simulink library "EOM"  (R2016b)
settings: Solver=VariableStepAuto  StartTime=0.0  StopTime=10.0  RelTol=1e-3
libraries: aerolib6dof2 x1
settings Model: Creator=Andrew  LastModifiedBy=Andrew

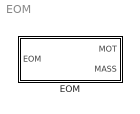
== system EOM ==
  EOM : Subsystem

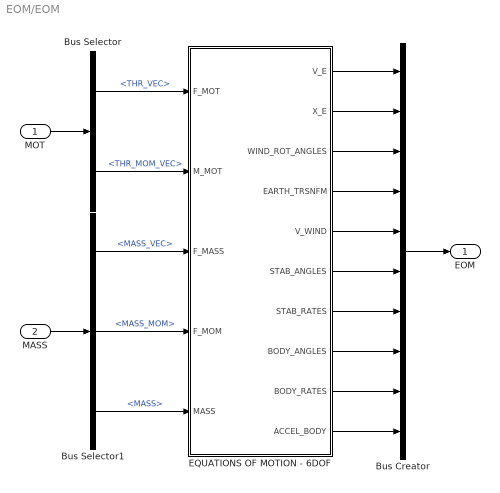
== system EOM/EOM ==
  MOT : Inport
  MASS : Inport  Port=2
  Bus Creator : BusCreator  Inputs=10
  Bus Selector : BusSelector  OutputSignals=THR_VEC,THR_MOM_VEC
  Bus Selector1 : BusSelector  OutputSignals=MASS_VEC,MASS_MOM,MASS
  EQUATIONS OF MOTION - 6DOF : Subsystem
  EOM : Outport
  wires:
  Bus Selector1/3 -> EQUATIONS OF MOTION - 6DOF/5(MASS)  "<MASS>"
  MOT/1 -> Bus Selector/1
  MASS/1 -> Bus Selector1/1
  Bus Selector/1 -> EQUATIONS OF MOTION - 6DOF/1(F_MOT)  "<THR_VEC>"
  Bus Selector/2 -> EQUATIONS OF MOTION - 6DOF/2(M_MOT)  "<THR_MOM_VEC>"
  Bus Selector1/1 -> EQUATIONS OF MOTION - 6DOF/3(F_MASS)  "<MASS_VEC>"
  Bus Selector1/2 -> EQUATIONS OF MOTION - 6DOF/4(F_MOM)  "<MASS_MOM>"
  EQUATIONS OF MOTION - 6DOF/7(STAB_RATES) -> Bus Creator/7
  EQUATIONS OF MOTION - 6DOF/6(STAB_ANGLES) -> Bus Creator/6
  EQUATIONS OF MOTION - 6DOF/5(V_WIND) -> Bus Creator/5
  EQUATIONS OF MOTION - 6DOF/1(V_E) -> Bus Creator/1
  EQUATIONS OF MOTION - 6DOF/8(BODY_ANGLES) -> Bus Creator/8
  EQUATIONS OF MOTION - 6DOF/4(EARTH_TRSNFM) -> Bus Creator/4
  EQUATIONS OF MOTION - 6DOF/3(WIND_ROT_ANGLES) -> Bus Creator/3
  EQUATIONS OF MOTION - 6DOF/10(ACCEL_BODY) -> Bus Creator/10
  EQUATIONS OF MOTION - 6DOF/2(X_E) -> Bus Creator/2
  EQUATIONS OF MOTION - 6DOF/9(BODY_RATES) -> Bus Creator/9
  Bus Creator/1 -> EOM/1

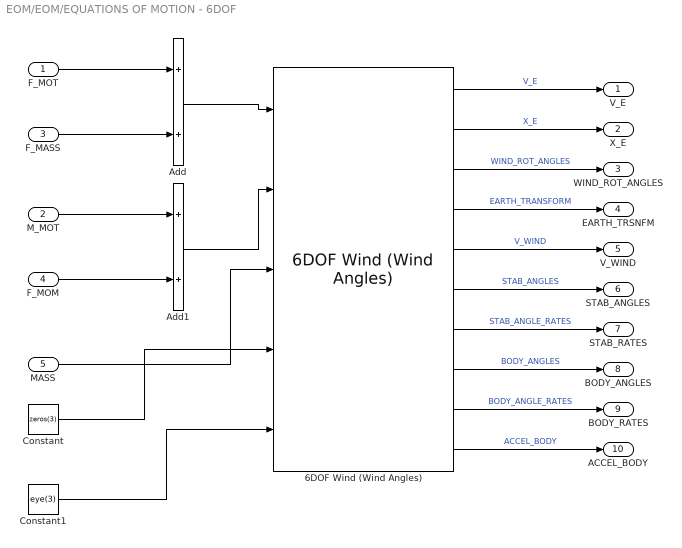
== system EOM/EOM/EQUATIONS OF MOTION - 6DOF ==
  F_MOT : Inport
  M_MOT : Inport  Port=2
  F_MASS : Inport  Port=3
  F_MOM : Inport  Port=4
  MASS : Inport  Port=5
  6DOF Wind (Wind Angles) : aerolib6dof2/6DOF Wind (Wind Angles)  units=English (Velocity in ft/s)  mtype=Custom Variable  rep=Wind Angles  xme_0=[0 0 -9]  Vm_0=[0.001 0 0]  wind_0=[0 0.5*pi 0]  pm_0=[0 0 0]  mass_0=0.0  mass_e=0.5  mass_f=2.0  inertia=eye(3)  inertia_e=eye(3)  inertia_f=2*eye(3)  vre_flag=off
  Add : Sum
  Add1 : Sum
  Constant : Constant  Value=zeros(3)  VectorParams1D=off
  Constant1 : Constant  Value=eye(3)  VectorParams1D=off
  V_E : Outport
  X_E : Outport  Port=2
  WIND_ROT_ANGLES : Outport  Port=3
  EARTH_TRSNFM : Outport  Port=4
  V_WIND : Outport  Port=5
  STAB_ANGLES : Outport  Port=6
  STAB_RATES : Outport  Port=7
  BODY_ANGLES : Outport  Port=8
  BODY_RATES : Outport  Port=9
  ACCEL_BODY : Outport  Port=10
  wires:
  F_MASS/1 -> Add/2
  Constant1/1 -> 6DOF Wind (Wind Angles)/5
  Constant/1 -> 6DOF Wind (Wind Angles)/4
  MASS/1 -> 6DOF Wind (Wind Angles)/3
  Add/1 -> 6DOF Wind (Wind Angles)/1
  Add1/1 -> 6DOF Wind (Wind Angles)/2
  F_MOT/1 -> Add/1
  M_MOT/1 -> Add1/1
  F_MOM/1 -> Add1/2
  6DOF Wind (Wind Angles)/1 -> V_E/1  "V_E"
  6DOF Wind (Wind Angles)/2 -> X_E/1  "X_E"
  6DOF Wind (Wind Angles)/3 -> WIND_ROT_ANGLES/1  "WIND_ROT_ANGLES"
  6DOF Wind (Wind Angles)/4 -> EARTH_TRSNFM/1  "EARTH_TRANSFORM"
  6DOF Wind (Wind Angles)/5 -> V_WIND/1  "V_WIND"
  6DOF Wind (Wind Angles)/6 -> STAB_ANGLES/1  "STAB_ANGLES"
  6DOF Wind (Wind Angles)/7 -> STAB_RATES/1  "STAB_ANGLE_RATES"
  6DOF Wind (Wind Angles)/8 -> BODY_ANGLES/1  "BODY_ANGLES"
  6DOF Wind (Wind Angles)/9 -> BODY_RATES/1  "BODY_ANGLE_RATES"
  6DOF Wind (Wind Angles)/10 -> ACCEL_BODY/1  "ACCEL_BODY"
